simulink model "ScenarioAnimation"  (R2020a)
settings: Solver=VariableStepAuto  StartTime=0.0  StopTime=15  RelTol=1e-3
InitFcn:
  | createDrivingScenario1();
libraries: drivinglib x2, drivingscenarioandsensors x2, sldrtlib x1
settings Model: PacingRate=0.320000  Creator=qihan  LastModifiedBy=qihan

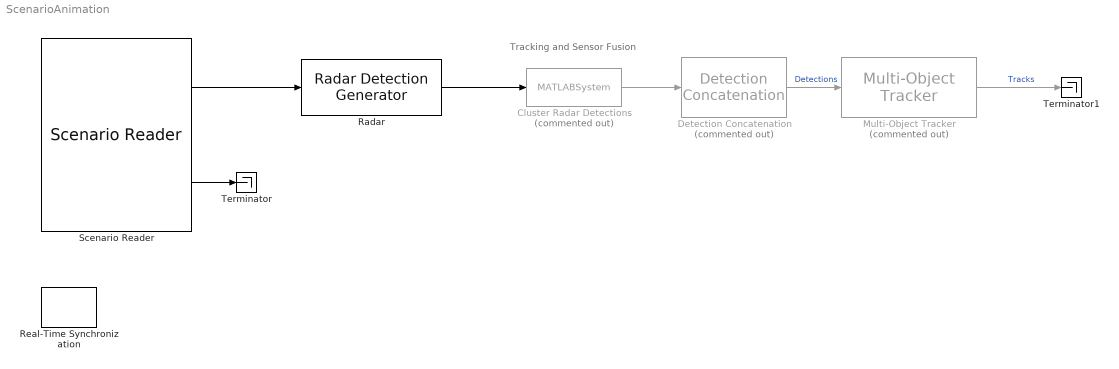
== system ScenarioAnimation ==
  note: Tracking and Sensor Fusion
  Cluster Radar Detections : MATLABSystem  Commented=on  System=helperClusterDetections  ClusterSize=5  BusNameSource=Auto  BusName=BusClusterDetections  SimulateUsing=Interpreted execution
      mask Type: helperClusterDetections
      mask Display:
      | disp(['Detection' char(10) 'Clustering']);
      | port_label('input',1,'In');
      | port_label('output',1,'Out');
  Detection Concatenation : drivinglib/Detection Concatenation  Commented=on  NumInputs=1  BusNameSource=Auto  BusName=BusDetectionConcatenation1  SimulateUsing=Interpreted execution
      settings: SourceProductBaseCode=DR
  Multi-Object Tracker : drivinglib/Multi-Object Tracker  Commented=on  TrackerIndex=uint32( 0 )  FilterInitializationFcn=helperInitSimulinkDemoFilter  AssignmentThreshold=50  ConfirmationThreshold=[ 2, 3 ]  DeletionThreshold=[5,5]  MaxNumTracks=20  MaxNumSensors=8  StateParams=struct  TimeInputSource=Auto  HasCostMatrixInput=off  HasDetectableTrackIDsInput=off  BusNameSource=Auto  BusName=BusMultiObjectTracker1  TentativeTracksOutputPort=off  AllTracksOutputPort=off  SimulateUsing=Interpreted execution
      settings: SourceProductBaseCode=DR
  Radar : drivingscenarioandsensors/Radar Detection Generator  SensorIndex=1  UpdateInterval=0.1  SensorLocation=[3.7 0]  Height=0.2  Yaw=0  Pitch=0  Roll=0  BusNameSource=Auto  BusName=BusRadarDetectionGenerator  MaxNumDetectionsSource=Property  MaxNumDetections=50  DetectionCoordinates=Ego Cartesian  SimulateUsing=Interpreted execution  AzimuthResolution=4  ElevationResolution=10  RangeResolution=2.5  RangeRateResolution=0.5  AzimuthBiasFraction=0.1  ElevationBiasFraction=0.1  RangeBiasFraction=0.05  RangeRateBiasFraction=0.05  FieldOfView=[20 5]  MaxRange=100  RangeRateLimits=[-100 100]  DetectionProbability=0.9  FalseAlarmRate=1e-06  ReferenceRange=100  ReferenceRCS=0  HasElevation=off  HasRangeRate=on  HasNoise=on  HasFalseAlarms=on  HasOcclusion=on  InitialSeedSource=Repeatable  InitialSeed=0  UsedSeed=0  ActorProfilesSource=MATLAB expression  ActorProfilesParameters=driving.internal.ActorProfilesRadarParameters  ActorProfilesExpression=[struct('ActorID',1,'ClassID',1,'Length',4.7,'Width',1.8,'Height',1.4,'OriginOffset',[-1.35 0 0],'MeshVertices',[3.7 -0.9 1.4;3.7 0.9 1.4;-1 0.9 1.4;-1 -0.9 1.4;3.7 -0.9 0;3.7 0.9 0;-1 0.9 0;-1 -0.9 0],'MeshFaces',[6 2 1;1 5 6;8 4 3;3 7 8;6 7 3;3 2 6;5 1 4;4 8 5;4 1 2;2 3 4;7 6 5;5 8 7],'RCSPattern',[10 10;10 10],'RCSAzimuthAngles',[-180 180],'RCSElevationAngles',[-90 90]); struct('ActorID',2,'ClassID',1,'Length',4.7,'Width',1.8,'Height',1.4,'OriginOffset',[-1.35 0 0],'MeshVertices',[3.7 -0.9 1.4;3.7 0.9 1.4;-1 0.9 1.4;-1 -0.9 1.4;3.7 -0.9 0;3.7 0.9 0;-1 0.9 0;-1 -0.9 0],'MeshFaces',[6 2 1;1 5 6;8 4 3;3 7 8;6 7 3;3 2 6;5 1 4;4 8 5;4 1 2;2 3 4;7 6 5;5 8 7],'RCSPattern',[10 10;10 10],'RCSAzimuthAngles',[-180 180],'RCSElevationAngles',[-90 90]); struct('ActorID',3,'ClassID',1,'Length',4.7,'Width',1.8,'Height',1.4,'OriginOffset',[-1.35 0 0],'MeshVertices',[3.7 -0.9 1.4;3.7 0.9 1.4;-1 0.9 1.4;-1 -0.9 1.4;3.7 -0.9 0;3.7 0.9 0;-1 0.9 0;-1 -0.9 0],'MeshFaces',[6 2 1;1 5 6;8 4 3;3 7 8;6 7 3;3 2 6;5 1 4;4 8 5;4 1 2;2 3 4;7 6 5;5 8 7],'RCSPattern',[10 10;10 10],'RCSAzimuthAngles',[-180 180],'RCSElevationAngles',[-90 90])]
      settings: SourceProductBaseCode=DR
  Real-Time Synchronization : sldrtlib/Real-Time Synchronization  SampleTime=0.1  MaxMissedTicks=10  ShowMissedTicks=off  YieldWhenWaiting=off
  Scenario Reader : drivingscenarioandsensors/Scenario Reader  ScenarioSource=From workspace  ScenarioFileName=C:\Users\qihan\Desktop\Git\Vehicle-following-model-with-3DAnimation\roads.mat  ScenarioVariableName=ans  OutputCoordinateSystem=Vehicle coordinates  EgoVehicleSource=Scenario  OrientVehiclesOnRoad=off  EgoVehicleActorID=1  OutputEgoVehiclePose=off  SampleTime=0.1  LaneBoundaryOutput=Ego vehicle lane boundaries  LaneBoundaryDistance=0:0.5:9.5  LaneBoundaryLocation=Center of lane markings  BusNameSource=Auto  BusName=BusActors  BusName2Source=Auto  BusName2=BusVision1  BusName3Source=Auto  BusName3=BusEgoActor  ShowCoordinateLabels=on  SimulateUsing=Interpreted execution
  Terminator : Terminator
  Terminator1 : Terminator
  wires:
  Radar/1 -> Cluster Radar Detections/1
  Detection Concatenation/1 -> Multi-Object Tracker/1  "Detections"
  Cluster Radar Detections/1 -> Detection Concatenation/1
  Multi-Object Tracker/1 -> Terminator1/1  "Tracks"
  Scenario Reader/1 -> Radar/1
  Scenario Reader/2 -> Terminator/1
